simulink model "LaptopTest"  (R2015b)
settings: Solver=VariableStepAuto  StartTime=0.0  StopTime=inf  RelTol=1e-3
libraries: aerolibanimutils x1, simulink x1, dspnetwork x1
(part 1 of 4)
settings Model: Creator=Ryuu  LastModifiedBy=Ryuu

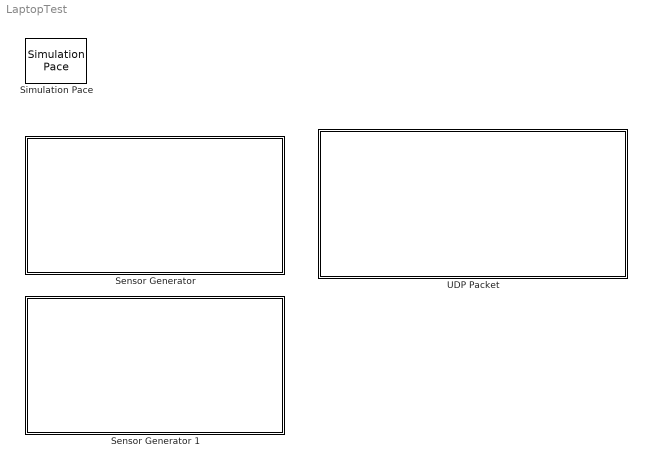
== system LaptopTest ==
  "Sensor Generator " : Subsystem
  Sensor Generator 1 : Subsystem
  Simulation Pace : aerolibanimutils/Simulation Pace  SimulationPace=1  SleepMode=MATLAB Thread  OutputPaceError=off  SampleTime=1/30
  UDP Packet : Subsystem

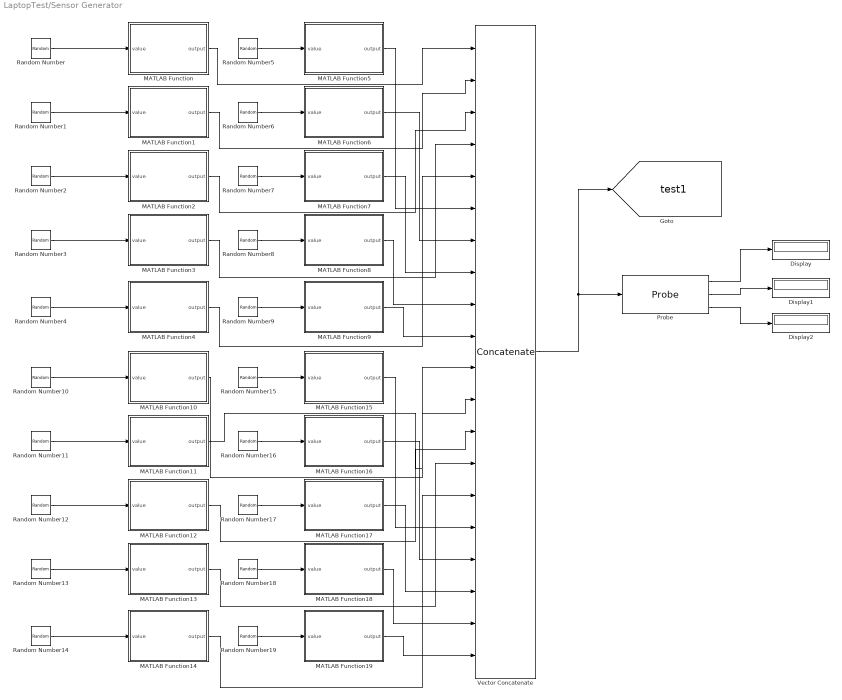
== system LaptopTest/Sensor Generator  ==
  Display : Display
  Display1 : Display
  Display2 : Display
  MATLAB Function : MATLAB Function  TreatAsAtomicUnit=on  mask(Signal Serializer){identifier=101}
      mask prompts: identifier "ID:"
      mask help:
      | Define and serialize a signal.
      |
      | The ID is the identifier of a signal.
      | - It must be unique.
      | - It must be numeric.
      | - It must match the ID defined for the signal on the GUI side.
  MATLAB Function1 : MATLAB Function  TreatAsAtomicUnit=on  mask(Signal Serializer){identifier=102}
      mask prompts: identifier "ID:"
      mask help:
      | Define and serialize a signal.
      |
      | The ID is the identifier of a signal.
      | - It must be unique.
      | - It must be numeric.
      | - It must match the ID defined for the signal on the GUI side.
  MATLAB Function10 : MATLAB Function  TreatAsAtomicUnit=on  mask(Signal Serializer){identifier=301}
      mask prompts: identifier "ID:"
      mask help:
      | Define and serialize a signal.
      |
      | The ID is the identifier of a signal.
      | - It must be unique.
      | - It must be numeric.
      | - It must match the ID defined for the signal on the GUI side.
  MATLAB Function11 : MATLAB Function  TreatAsAtomicUnit=on  mask(Signal Serializer){identifier=302}
      mask prompts: identifier "ID:"
      mask help:
      | Define and serialize a signal.
      |
      | The ID is the identifier of a signal.
      | - It must be unique.
      | - It must be numeric.
      | - It must match the ID defined for the signal on the GUI side.
  MATLAB Function12 : MATLAB Function  TreatAsAtomicUnit=on  mask(Signal Serializer){identifier=303}
      mask prompts: identifier "ID:"
      mask help:
      | Define and serialize a signal.
      |
      | The ID is the identifier of a signal.
      | - It must be unique.
      | - It must be numeric.
      | - It must match the ID defined for the signal on the GUI side.
  MATLAB Function13 : MATLAB Function  TreatAsAtomicUnit=on  mask(Signal Serializer){identifier=304}
      mask prompts: identifier "ID:"
      mask help:
      | Define and serialize a signal.
      |
      | The ID is the identifier of a signal.
      | - It must be unique.
      | - It must be numeric.
      | - It must match the ID defined for the signal on the GUI side.
  MATLAB Function14 : MATLAB Function  TreatAsAtomicUnit=on  mask(Signal Serializer){identifier=305}
      mask prompts: identifier "ID:"
      mask help:
      | Define and serialize a signal.
      |
      | The ID is the identifier of a signal.
      | - It must be unique.
      | - It must be numeric.
      | - It must match the ID defined for the signal on the GUI side.
  MATLAB Function15 : MATLAB Function  TreatAsAtomicUnit=on  mask(Signal Serializer){identifier=401}
      mask prompts: identifier "ID:"
      mask help:
      | Define and serialize a signal.
      |
      | The ID is the identifier of a signal.
      | - It must be unique.
      | - It must be numeric.
      | - It must match the ID defined for the signal on the GUI side.
  MATLAB Function16 : MATLAB Function  TreatAsAtomicUnit=on  mask(Signal Serializer){identifier=402}
      mask prompts: identifier "ID:"
      mask help:
      | Define and serialize a signal.
      |
      | The ID is the identifier of a signal.
      | - It must be unique.
      | - It must be numeric.
      | - It must match the ID defined for the signal on the GUI side.
  MATLAB Function17 : MATLAB Function  TreatAsAtomicUnit=on  mask(Signal Serializer){identifier=403}
      mask prompts: identifier "ID:"
      mask help:
      | Define and serialize a signal.
      |
      | The ID is the identifier of a signal.
      | - It must be unique.
      | - It must be numeric.
      | - It must match the ID defined for the signal on the GUI side.
  MATLAB Function18 : MATLAB Function  TreatAsAtomicUnit=on  mask(Signal Serializer){identifier=404}
      mask prompts: identifier "ID:"
      mask help:
      | Define and serialize a signal.
      |
      | The ID is the identifier of a signal.
      | - It must be unique.
      | - It must be numeric.
      | - It must match the ID defined for the signal on the GUI side.
  MATLAB Function19 : MATLAB Function  TreatAsAtomicUnit=on  mask(Signal Serializer){identifier=405}
      mask prompts: identifier "ID:"
      mask help:
      | Define and serialize a signal.
      |
      | The ID is the identifier of a signal.
      | - It must be unique.
      | - It must be numeric.
      | - It must match the ID defined for the signal on the GUI side.
  MATLAB Function2 : MATLAB Function  TreatAsAtomicUnit=on  mask(Signal Serializer){identifier=103}
      mask prompts: identifier "ID:"
      mask help:
      | Define and serialize a signal.
      |
      | The ID is the identifier of a signal.
      | - It must be unique.
      | - It must be numeric.
      | - It must match the ID defined for the signal on the GUI side.
  MATLAB Function3 : MATLAB Function  TreatAsAtomicUnit=on  mask(Signal Serializer){identifier=104}
      mask prompts: identifier "ID:"
      mask help:
      | Define and serialize a signal.
      |
      | The ID is the identifier of a signal.
      | - It must be unique.
      | - It must be numeric.
      | - It must match the ID defined for the signal on the GUI side.
  MATLAB Function4 : MATLAB Function  TreatAsAtomicUnit=on  mask(Signal Serializer){identifier=105}
      mask prompts: identifier "ID:"
      mask help:
      | Define and serialize a signal.
      |
      | The ID is the identifier of a signal.
      | - It must be unique.
      | - It must be numeric.
      | - It must match the ID defined for the signal on the GUI side.
  MATLAB Function5 : MATLAB Function  TreatAsAtomicUnit=on  mask(Signal Serializer){identifier=201}
      mask prompts: identifier "ID:"
      mask help:
      | Define and serialize a signal.
      |
      | The ID is the identifier of a signal.
      | - It must be unique.
      | - It must be numeric.
      | - It must match the ID defined for the signal on the GUI side.
  MATLAB Function6 : MATLAB Function  TreatAsAtomicUnit=on  mask(Signal Serializer){identifier=202}
      mask prompts: identifier "ID:"
      mask help:
      | Define and serialize a signal.
      |
      | The ID is the identifier of a signal.
      | - It must be unique.
      | - It must be numeric.
      | - It must match the ID defined for the signal on the GUI side.
  MATLAB Function7 : MATLAB Function  TreatAsAtomicUnit=on  mask(Signal Serializer){identifier=203}
      mask prompts: identifier "ID:"
      mask help:
      | Define and serialize a signal.
      |
      | The ID is the identifier of a signal.
      | - It must be unique.
      | - It must be numeric.
      | - It must match the ID defined for the signal on the GUI side.
  MATLAB Function8 : MATLAB Function  TreatAsAtomicUnit=on  mask(Signal Serializer){identifier=204}
      mask prompts: identifier "ID:"
      mask help:
      | Define and serialize a signal.
      |
      | The ID is the identifier of a signal.
      | - It must be unique.
      | - It must be numeric.
      | - It must match the ID defined for the signal on the GUI side.
  MATLAB Function9 : MATLAB Function  TreatAsAtomicUnit=on  mask(Signal Serializer){identifier=205}
      mask prompts: identifier "ID:"
      mask help:
      | Define and serialize a signal.
      |
      | The ID is the identifier of a signal.
      | - It must be unique.
      | - It must be numeric.
      | - It must match the ID defined for the signal on the GUI side.
  Probe : Probe  ProbeComplexSignal=off  ProbeSignalDimensions=on
  Random Number : RandomNumber  Mean=100  Variance=50  Seed=101  SampleTime=0.02
  Random Number1 : RandomNumber  Mean=100  Variance=50  Seed=102  SampleTime=0.02
  Random Number10 : RandomNumber  Mean=100  Variance=50  Seed=301  SampleTime=0.02
  Random Number11 : RandomNumber  Mean=100  Variance=50  Seed=302  SampleTime=0.02
  Random Number12 : RandomNumber  Mean=100  Variance=50  Seed=303  SampleTime=0.02
  Random Number13 : RandomNumber  Mean=100  Variance=50  Seed=304  SampleTime=0.02
  Random Number14 : RandomNumber  Mean=100  Variance=50  Seed=305  SampleTime=0.02
  Random Number15 : RandomNumber  Mean=100  Variance=50  Seed=401  SampleTime=0.02
  Random Number16 : RandomNumber  Mean=100  Variance=50  Seed=402  SampleTime=0.02
  Random Number17 : RandomNumber  Mean=100  Variance=50  Seed=403  SampleTime=0.02
  Random Number18 : RandomNumber  Mean=100  Variance=50  Seed=404  SampleTime=0.02
  Random Number19 : RandomNumber  Mean=100  Variance=50  Seed=405  SampleTime=0.02
  Random Number2 : RandomNumber  Mean=100  Variance=50  Seed=103  SampleTime=0.02
  Random Number3 : RandomNumber  Mean=100  Variance=50  Seed=104  SampleTime=0.02
  Random Number4 : RandomNumber  Mean=100  Variance=50  Seed=105  SampleTime=0.02
  Random Number5 : RandomNumber  Mean=100  Variance=50  Seed=201  SampleTime=0.02
  Random Number6 : RandomNumber  Mean=100  Variance=50  Seed=202  SampleTime=0.02
  Random Number7 : RandomNumber  Mean=100  Variance=50  Seed=203  SampleTime=0.02
  Random Number8 : RandomNumber  Mean=100  Variance=50  Seed=204  SampleTime=0.02
  Random Number9 : RandomNumber  Mean=100  Variance=50  Seed=205  SampleTime=0.02
  Vector Concatenate : Concatenate  NumInputs=20
  tag scope: test1=global
  wires:
  MATLAB Function/1(output) -> Vector Concatenate/1
  Random Number2/1 -> MATLAB Function2/1(value)
  Random Number3/1 -> MATLAB Function3/1(value)
  Random Number4/1 -> MATLAB Function4/1(value)
  Random Number5/1 -> MATLAB Function5/1(value)
  Random Number6/1 -> MATLAB Function6/1(value)
  Random Number7/1 -> MATLAB Function7/1(value)
  Random Number8/1 -> MATLAB Function8/1(value)
  Random Number9/1 -> MATLAB Function9/1(value)
  MATLAB Function1/1(output) -> Vector Concatenate/2
  MATLAB Function2/1(output) -> Vector Concatenate/3
  MATLAB Function3/1(output) -> Vector Concatenate/4
  MATLAB Function4/1(output) -> Vector Concatenate/5
  MATLAB Function5/1(output) -> Vector Concatenate/6
  MATLAB Function6/1(output) -> Vector Concatenate/7
  MATLAB Function8/1(output) -> Vector Concatenate/9
  MATLAB Function7/1(output) -> Vector Concatenate/8
  MATLAB Function9/1(output) -> Vector Concatenate/10
  Random Number/1 -> MATLAB Function/1(value)
  Random Number1/1 -> MATLAB Function1/1(value)
  Vector Concatenate/1 -> [test1], Probe/1
  Probe/1 -> Display/1
  Probe/2 -> Display1/1
  Probe/3 -> Display2/1
  MATLAB Function10/1(output) -> Vector Concatenate/11
  Random Number12/1 -> MATLAB Function12/1(value)
  Random Number13/1 -> MATLAB Function13/1(value)
  Random Number14/1 -> MATLAB Function14/1(value)
  Random Number15/1 -> MATLAB Function15/1(value)
  Random Number16/1 -> MATLAB Function16/1(value)
  Random Number17/1 -> MATLAB Function17/1(value)
  Random Number18/1 -> MATLAB Function18/1(value)
  Random Number19/1 -> MATLAB Function19/1(value)
  MATLAB Function11/1(output) -> Vector Concatenate/12
  MATLAB Function12/1(output) -> Vector Concatenate/13
  MATLAB Function13/1(output) -> Vector Concatenate/14
  MATLAB Function14/1(output) -> Vector Concatenate/15
  MATLAB Function15/1(output) -> Vector Concatenate/16
  MATLAB Function16/1(output) -> Vector Concatenate/17
  MATLAB Function18/1(output) -> Vector Concatenate/19
  MATLAB Function17/1(output) -> Vector Concatenate/18
  MATLAB Function19/1(output) -> Vector Concatenate/20
  Random Number10/1 -> MATLAB Function10/1(value)
  Random Number11/1 -> MATLAB Function11/1(value)

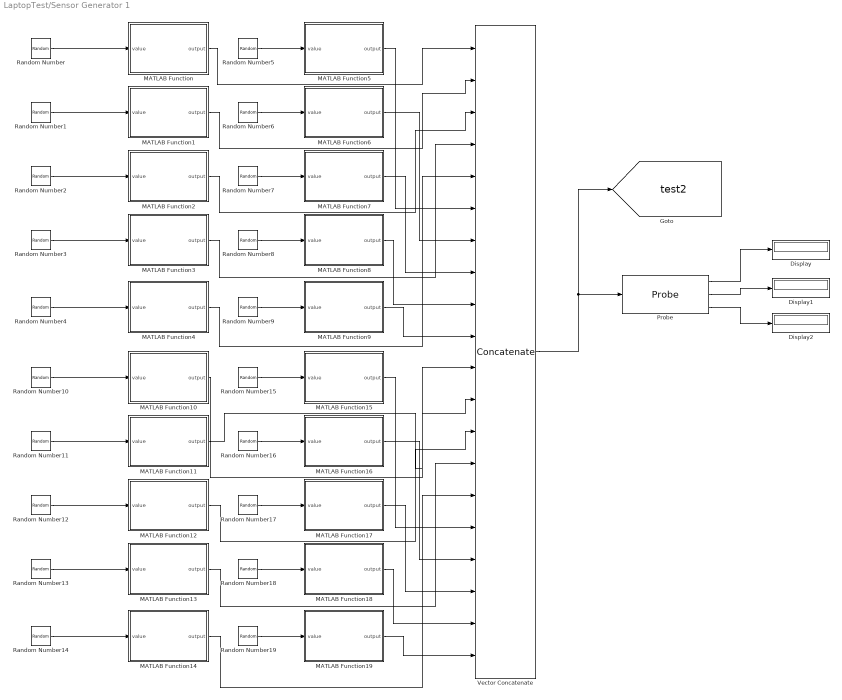
== system LaptopTest/Sensor Generator 1 ==
  Display : Display
  Display1 : Display
  Display2 : Display
  MATLAB Function : MATLAB Function  TreatAsAtomicUnit=on  mask(Signal Serializer){identifier=501}
      mask prompts: identifier "ID:"
      mask help:
      | Define and serialize a signal.
      |
      | The ID is the identifier of a signal.
      | - It must be unique.
      | - It must be numeric.
      | - It must match the ID defined for the signal on the GUI side.
  MATLAB Function1 : MATLAB Function  TreatAsAtomicUnit=on  mask(Signal Serializer){identifier=502}
      mask prompts: identifier "ID:"
      mask help:
      | Define and serialize a signal.
      |
      | The ID is the identifier of a signal.
      | - It must be unique.
      | - It must be numeric.
      | - It must match the ID defined for the signal on the GUI side.
  MATLAB Function10 : MATLAB Function  TreatAsAtomicUnit=on  mask(Signal Serializer){identifier=701}
      mask prompts: identifier "ID:"
      mask help:
      | Define and serialize a signal.
      |
      | The ID is the identifier of a signal.
      | - It must be unique.
      | - It must be numeric.
      | - It must match the ID defined for the signal on the GUI side.
  MATLAB Function11 : MATLAB Function  TreatAsAtomicUnit=on  mask(Signal Serializer){identifier=702}
      mask prompts: identifier "ID:"
      mask help:
      | Define and serialize a signal.
      |
      | The ID is the identifier of a signal.
      | - It must be unique.
      | - It must be numeric.
      | - It must match the ID defined for the signal on the GUI side.
  MATLAB Function12 : MATLAB Function  TreatAsAtomicUnit=on  mask(Signal Serializer){identifier=703}
      mask prompts: identifier "ID:"
      mask help:
      | Define and serialize a signal.
      |
      | The ID is the identifier of a signal.
      | - It must be unique.
      | - It must be numeric.
      | - It must match the ID defined for the signal on the GUI side.
  MATLAB Function13 : MATLAB Function  TreatAsAtomicUnit=on  mask(Signal Serializer){identifier=704}
      mask prompts: identifier "ID:"
      mask help:
      | Define and serialize a signal.
      |
      | The ID is the identifier of a signal.
      | - It must be unique.
      | - It must be numeric.
      | - It must match the ID defined for the signal on the GUI side.
  MATLAB Function14 : MATLAB Function  TreatAsAtomicUnit=on  mask(Signal Serializer){identifier=705}
      mask prompts: identifier "ID:"
      mask help:
      | Define and serialize a signal.
      |
      | The ID is the identifier of a signal.
      | - It must be unique.
      | - It must be numeric.
      | - It must match the ID defined for the signal on the GUI side.
  MATLAB Function15 : MATLAB Function  TreatAsAtomicUnit=on  mask(Signal Serializer){identifier=801}
      mask prompts: identifier "ID:"
      mask help:
      | Define and serialize a signal.
      |
      | The ID is the identifier of a signal.
      | - It must be unique.
      | - It must be numeric.
      | - It must match the ID defined for the signal on the GUI side.
  MATLAB Function16 : MATLAB Function  TreatAsAtomicUnit=on  mask(Signal Serializer){identifier=802}
      mask prompts: identifier "ID:"
      mask help:
      | Define and serialize a signal.
      |
      | The ID is the identifier of a signal.
      | - It must be unique.
      | - It must be numeric.
      | - It must match the ID defined for the signal on the GUI side.
  MATLAB Function17 : MATLAB Function  TreatAsAtomicUnit=on  mask(Signal Serializer){identifier=803}
      mask prompts: identifier "ID:"
      mask help:
      | Define and serialize a signal.
      |
      | The ID is the identifier of a signal.
      | - It must be unique.
      | - It must be numeric.
      | - It must match the ID defined for the signal on the GUI side.
  MATLAB Function18 : MATLAB Function  TreatAsAtomicUnit=on  mask(Signal Serializer){identifier=804}
      mask prompts: identifier "ID:"
      mask help:
      | Define and serialize a signal.
      |
      | The ID is the identifier of a signal.
      | - It must be unique.
      | - It must be numeric.
      | - It must match the ID defined for the signal on the GUI side.
  MATLAB Function19 : MATLAB Function  TreatAsAtomicUnit=on  mask(Signal Serializer){identifier=805}
      mask prompts: identifier "ID:"
      mask help:
      | Define and serialize a signal.
      |
      | The ID is the identifier of a signal.
      | - It must be unique.
      | - It must be numeric.
      | - It must match the ID defined for the signal on the GUI side.
  MATLAB Function2 : MATLAB Function  TreatAsAtomicUnit=on  mask(Signal Serializer){identifier=503}
      mask prompts: identifier "ID:"
      mask help:
      | Define and serialize a signal.
      |
      | The ID is the identifier of a signal.
      | - It must be unique.
      | - It must be numeric.
      | - It must match the ID defined for the signal on the GUI side.
  MATLAB Function3 : MATLAB Function  TreatAsAtomicUnit=on  mask(Signal Serializer){identifier=504}
      mask prompts: identifier "ID:"
      mask help:
      | Define and serialize a signal.
      |
      | The ID is the identifier of a signal.
      | - It must be unique.
      | - It must be numeric.
      | - It must match the ID defined for the signal on the GUI side.
  MATLAB Function4 : MATLAB Function  TreatAsAtomicUnit=on  mask(Signal Serializer){identifier=505}
      mask prompts: identifier "ID:"
      mask help:
      | Define and serialize a signal.
      |
      | The ID is the identifier of a signal.
      | - It must be unique.
      | - It must be numeric.
      | - It must match the ID defined for the signal on the GUI side.
  MATLAB Function5 : MATLAB Function  TreatAsAtomicUnit=on  mask(Signal Serializer){identifier=601}
      mask prompts: identifier "ID:"
      mask help:
      | Define and serialize a signal.
      |
      | The ID is the identifier of a signal.
      | - It must be unique.
      | - It must be numeric.
      | - It must match the ID defined for the signal on the GUI side.
  MATLAB Function6 : MATLAB Function  TreatAsAtomicUnit=on  mask(Signal Serializer){identifier=602}
      mask prompts: identifier "ID:"
      mask help:
      | Define and serialize a signal.
      |
      | The ID is the identifier of a signal.
      | - It must be unique.
      | - It must be numeric.
      | - It must match the ID defined for the signal on the GUI side.
  MATLAB Function7 : MATLAB Function  TreatAsAtomicUnit=on  mask(Signal Serializer){identifier=603}
      mask prompts: identifier "ID:"
      mask help:
      | Define and serialize a signal.
      |
      | The ID is the identifier of a signal.
      | - It must be unique.
      | - It must be numeric.
      | - It must match the ID defined for the signal on the GUI side.
  MATLAB Function8 : MATLAB Function  TreatAsAtomicUnit=on  mask(Signal Serializer){identifier=604}
      mask prompts: identifier "ID:"
      mask help:
      | Define and serialize a signal.
      |
      | The ID is the identifier of a signal.
      | - It must be unique.
      | - It must be numeric.
      | - It must match the ID defined for the signal on the GUI side.
  MATLAB Function9 : MATLAB Function  TreatAsAtomicUnit=on  mask(Signal Serializer){identifier=605}
      mask prompts: identifier "ID:"
      mask help:
      | Define and serialize a signal.
      |
      | The ID is the identifier of a signal.
      | - It must be unique.
      | - It must be numeric.
      | - It must match the ID defined for the signal on the GUI side.
  Probe : Probe  ProbeComplexSignal=off  ProbeSignalDimensions=on
  Random Number : RandomNumber  Mean=100  Variance=50  Seed=501  SampleTime=0.02
  Random Number1 : RandomNumber  Mean=100  Variance=50  Seed=502  SampleTime=0.02
  Random Number10 : RandomNumber  Mean=100  Variance=50  Seed=701  SampleTime=0.02
  Random Number11 : RandomNumber  Mean=100  Variance=50  Seed=702  SampleTime=0.02
  Random Number12 : RandomNumber  Mean=100  Variance=50  Seed=703  SampleTime=0.02
  Random Number13 : RandomNumber  Mean=100  Variance=50  Seed=704  SampleTime=0.02
  Random Number14 : RandomNumber  Mean=100  Variance=50  Seed=705  SampleTime=0.02
  Random Number15 : RandomNumber  Mean=100  Variance=50  Seed=801  SampleTime=0.02
  Random Number16 : RandomNumber  Mean=100  Variance=50  Seed=802  SampleTime=0.02
  Random Number17 : RandomNumber  Mean=100  Variance=50  Seed=803  SampleTime=0.02
  Random Number18 : RandomNumber  Mean=100  Variance=50  Seed=804  SampleTime=0.02
  Random Number19 : RandomNumber  Mean=100  Variance=50  Seed=805  SampleTime=0.02
  Random Number2 : RandomNumber  Mean=100  Variance=50  Seed=503  SampleTime=0.02
  Random Number3 : RandomNumber  Mean=100  Variance=50  Seed=504  SampleTime=0.02
  Random Number4 : RandomNumber  Mean=100  Variance=50  Seed=505  SampleTime=0.02
  Random Number5 : RandomNumber  Mean=100  Variance=50  Seed=601  SampleTime=0.02
  Random Number6 : RandomNumber  Mean=100  Variance=50  Seed=602  SampleTime=0.02
  Random Number7 : RandomNumber  Mean=100  Variance=50  Seed=603  SampleTime=0.02
  Random Number8 : RandomNumber  Mean=100  Variance=50  Seed=604  SampleTime=0.02
  Random Number9 : RandomNumber  Mean=100  Variance=50  Seed=605  SampleTime=0.02
  Vector Concatenate : Concatenate  NumInputs=20
  tag scope: test2=global
  wires:
  MATLAB Function/1(output) -> Vector Concatenate/1
  Random Number2/1 -> MATLAB Function2/1(value)
  Random Number3/1 -> MATLAB Function3/1(value)
  Random Number4/1 -> MATLAB Function4/1(value)
  Random Number5/1 -> MATLAB Function5/1(value)
  Random Number6/1 -> MATLAB Function6/1(value)
  Random Number7/1 -> MATLAB Function7/1(value)
  Random Number8/1 -> MATLAB Function8/1(value)
  Random Number9/1 -> MATLAB Function9/1(value)
  MATLAB Function1/1(output) -> Vector Concatenate/2
  MATLAB Function2/1(output) -> Vector Concatenate/3
  MATLAB Function3/1(output) -> Vector Concatenate/4
  MATLAB Function4/1(output) -> Vector Concatenate/5
  MATLAB Function5/1(output) -> Vector Concatenate/6
  MATLAB Function6/1(output) -> Vector Concatenate/7
  MATLAB Function8/1(output) -> Vector Concatenate/9
  MATLAB Function7/1(output) -> Vector Concatenate/8
  MATLAB Function9/1(output) -> Vector Concatenate/10
  Random Number/1 -> MATLAB Function/1(value)
  Random Number1/1 -> MATLAB Function1/1(value)
  Vector Concatenate/1 -> [test2], Probe/1
  Probe/1 -> Display/1
  Probe/2 -> Display1/1
  Probe/3 -> Display2/1
  MATLAB Function10/1(output) -> Vector Concatenate/11
  Random Number12/1 -> MATLAB Function12/1(value)
  Random Number13/1 -> MATLAB Function13/1(value)
  Random Number14/1 -> MATLAB Function14/1(value)
  Random Number15/1 -> MATLAB Function15/1(value)
  Random Number16/1 -> MATLAB Function16/1(value)
  Random Number17/1 -> MATLAB Function17/1(value)
  Random Number18/1 -> MATLAB Function18/1(value)
  Random Number19/1 -> MATLAB Function19/1(value)
  MATLAB Function11/1(output) -> Vector Concatenate/12
  MATLAB Function12/1(output) -> Vector Concatenate/13
  MATLAB Function13/1(output) -> Vector Concatenate/14
  MATLAB Function14/1(output) -> Vector Concatenate/15
  MATLAB Function15/1(output) -> Vector Concatenate/16
  MATLAB Function16/1(output) -> Vector Concatenate/17
  MATLAB Function18/1(output) -> Vector Concatenate/19
  MATLAB Function17/1(output) -> Vector Concatenate/18
  MATLAB Function19/1(output) -> Vector Concatenate/20
  Random Number10/1 -> MATLAB Function10/1(value)
  Random Number11/1 -> MATLAB Function11/1(value)

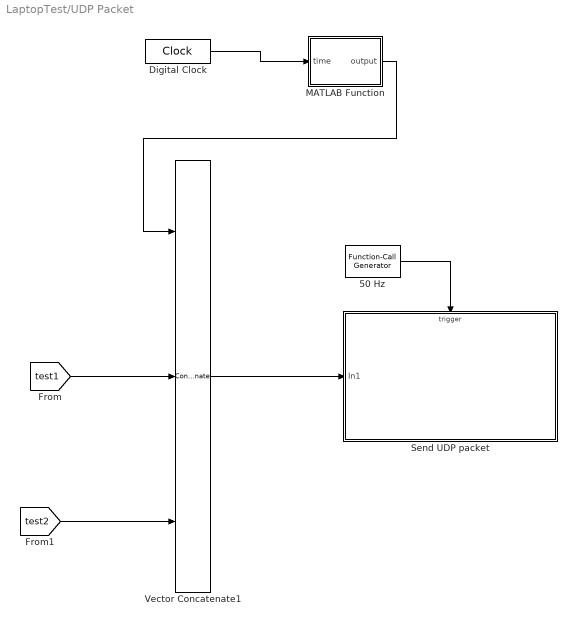
== system LaptopTest/UDP Packet ==
  50 Hz : simulink/Ports & Subsystems/Function-Call Generator  sample_time=0.02  numberOfIterations=1
  Digital Clock : DigitalClock  SampleTime=0.001
  MATLAB Function : MATLAB Function  TreatAsAtomicUnit=on
  Send UDP packet : Subsystem
  Vector Concatenate1 : Concatenate  NumInputs=3
  wires:
  [test1] -> Vector Concatenate1/2
  50 Hz/1 -> Send UDP packet/Trigger
  Vector Concatenate1/1 -> Send UDP packet/1(In1)
  Digital Clock/1 -> MATLAB Function/1(time)
  MATLAB Function/1(output) -> Vector Concatenate1/1
  [test2] -> Vector Concatenate1/3

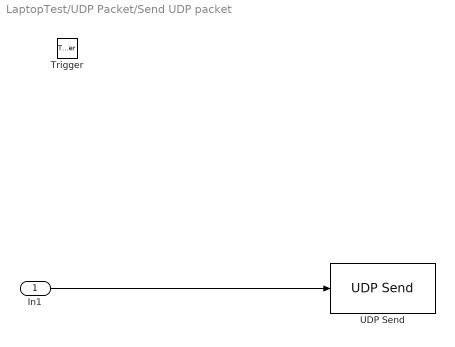
== system LaptopTest/UDP Packet/Send UDP packet ==
  In1 : Inport
  Trigger : TriggerPort  TriggerType=function-call  PortDimensions=1
  UDP Send : dspnetwork/UDP Send  remoteURL='192.168.21.1'  remotePort=25000  localURL='0.0.0.0'  localPortSource=Automatically determine  localPort=-1  sampletime=-1  separateLengthPort=0
  wires:
  In1/1 -> UDP Send/1

== matlab function LaptopTest/Sensor Generator /MATLAB Function1 ==
  data: value input; output output uint8 size=18; identifier parameter double
function output = data_serialize(value, identifier)

id_ser = sensor_serialize(identifier);
value_ser = sensor_serialize(value);

output = [
    id_ser;
    value_ser;
    ];
end


function m = sensor_serialize(v)
    % dispatch according to type
    if isnumeric(v) 
        m = serialize_numeric(v);
    elseif ischar(v)
        m = serialize_string(v);
    elseif islogical(v)
        m = serialize_logical(v);
	else
		error('Unsupported data type');
    end
end

% single scalar
function m = serialize_scalar(v)
    % Data type & data
    m = [class2tag(class(v)); typecast(v,'uint8').'];
end

% char arrays
function m = serialize_string(v)
    if size(v,1) == 1
        % horizontal string: Type, Length, and Data
        m = [uint8(0); typecast(uint32(length(v)),'uint8').'; uint8(v(:))];
    elseif sum(size(v)) == 0
        % '': special encoding
        m = uint8(200);
    else
        % general char array: Tag & Number of dimensions, Dimensions, Data
        m = [uint8(132); ndims(v); typecast(uint32(size(v)),'uint8').'; uint8(v(:))];
    end
end

% logical arrays
function m = serialize_logical(v)
    % Tag & Number of dimensions, Dimensions, Data
    m = [uint8(133); ndims(v); typecast(uint32(size(v)),'uint8').'; uint8(v(:))];
end

% non-complex and non-sparse numerical matrix
function m = serialize_numeric_simple(v)
    % Tag & Number of dimensions, Dimensions, Data
    m = [16+class2tag(class(v)); ndims(v); typecast(uint32(size(v)),'uint8').'; typecast(v(:).','uint8').'];
end

% Numeric Matrix: can be real/complex, sparse/full, scalar
function m = serialize_numeric(v)
    if issparse(v)
        % Data Type & Dimensions
        m = [uint8(130); typecast(uint64(size(v,1)), 'uint8').'; typecast(uint64(size(v,2)), 'uint8').']; % vectorize
        % Index vectors
        [i,j,s] = find(v);        
        % Real/Complex
        if isreal(v)
            m = [m; serialize_numeric_simple(i); serialize_numeric_simple(j); 1; serialize_numeric_simple(s)];
        else
            m = [m; serialize_numeric_simple(i); serialize_numeric_simple(j); 0; serialize_numeric_simple(real(s)); serialize_numeric_simple(imag(s))];
        end
    elseif ~isreal(v)
        % Data type & contents
        m = [uint8(131); serialize_numeric_simple(real(v)); serialize_numeric_simple(imag(v))];
    elseif isscalar(v)
        % Scalar
        m = serialize_scalar(v);
    else
        % Simple matrix
        m = serialize_numeric_simple(v);
    end
end

% *container* class to byte
function b = class2tag(cls)
	switch cls
		case 'string'
            b = uint8(0);
		case 'double'
			b = uint8(1);
		case 'single'
			b = uint8(2);
		case 'int8'
			b = uint8(3);
		case 'uint8'
			b = uint8(4);
		case 'int16'
			b = uint8(5);
		case 'uint16'
			b = uint8(6);
		case 'int32'
			b = uint8(7);
		case 'uint32'
			b = uint8(8);
		case 'int64'
			b = uint8(9);
		case 'uint64'
			b = uint8(10);
		otherwise
			error('Unknown class');
    end
end

== matlab function LaptopTest/Sensor Generator /MATLAB Function ==
  data: value input; output output uint8 size=18; identifier parameter double
function output = data_serialize(value, identifier)

id_ser = sensor_serialize(identifier);
value_ser = sensor_serialize(value);

output = [
    id_ser;
    value_ser;
    ];
end


function m = sensor_serialize(v)
    % dispatch according to type
    if isnumeric(v) 
        m = serialize_numeric(v);
    elseif ischar(v)
        m = serialize_string(v);
    elseif islogical(v)
        m = serialize_logical(v);
	else
		error('Unsupported data type');
    end
end

% single scalar
function m = serialize_scalar(v)
    % Data type & data
    m = [class2tag(class(v)); typecast(v,'uint8').'];
end

% char arrays
function m = serialize_string(v)
    if size(v,1) == 1
        % horizontal string: Type, Length, and Data
        m = [uint8(0); typecast(uint32(length(v)),'uint8').'; uint8(v(:))];
    elseif sum(size(v)) == 0
        % '': special encoding
        m = uint8(200);
    else
        % general char array: Tag & Number of dimensions, Dimensions, Data
        m = [uint8(132); ndims(v); typecast(uint32(size(v)),'uint8').'; uint8(v(:))];
    end
end

% logical arrays
function m = serialize_logical(v)
    % Tag & Number of dimensions, Dimensions, Data
    m = [uint8(133); ndims(v); typecast(uint32(size(v)),'uint8').'; uint8(v(:))];
end

% non-complex and non-sparse numerical matrix
function m = serialize_numeric_simple(v)
    % Tag & Number of dimensions, Dimensions, Data
    m = [16+class2tag(class(v)); ndims(v); typecast(uint32(size(v)),'uint8').'; typecast(v(:).','uint8').'];
end

% Numeric Matrix: can be real/complex, sparse/full, scalar
function m = serialize_numeric(v)
    if issparse(v)
        % Data Type & Dimensions
        m = [uint8(130); typecast(uint64(size(v,1)), 'uint8').'; typecast(uint64(size(v,2)), 'uint8').']; % vectorize
        % Index vectors
        [i,j,s] = find(v);        
        % Real/Complex
        if isreal(v)
            m = [m; serialize_numeric_simple(i); serialize_numeric_simple(j); 1; serialize_numeric_simple(s)];
        else
            m = [m; serialize_numeric_simple(i); serialize_numeric_simple(j); 0; serialize_numeric_simple(real(s)); serialize_numeric_simple(imag(s))];
        end
    elseif ~isreal(v)
        % Data type & contents
        m = [uint8(131); serialize_numeric_simple(real(v)); serialize_numeric_simple(imag(v))];
    elseif isscalar(v)
        % Scalar
        m = serialize_scalar(v);
    else
        % Simple matrix
        m = serialize_numeric_simple(v);
    end
end

% *container* class to byte
function b = class2tag(cls)
	switch cls
		case 'string'
            b = uint8(0);
		case 'double'
			b = uint8(1);
		case 'single'
			b = uint8(2);
		case 'int8'
			b = uint8(3);
		case 'uint8'
			b = uint8(4);
		case 'int16'
			b = uint8(5);
		case 'uint16'
			b = uint8(6);
		case 'int32'
			b = uint8(7);
		case 'uint32'
			b = uint8(8);
		case 'int64'
			b = uint8(9);
		case 'uint64'
			b = uint8(10);
		otherwise
			error('Unknown class');
    end
end

== matlab function LaptopTest/Sensor Generator /MATLAB Function2 ==
  data: value input; output output uint8 size=18; identifier parameter double
function output = data_serialize(value, identifier)

id_ser = sensor_serialize(identifier);
value_ser = sensor_serialize(value);

output = [
    id_ser;
    value_ser;
    ];
end


function m = sensor_serialize(v)
    % dispatch according to type
    if isnumeric(v) 
        m = serialize_numeric(v);
    elseif ischar(v)
        m = serialize_string(v);
    elseif islogical(v)
        m = serialize_logical(v);
	else
		error('Unsupported data type');
    end
end

% single scalar
function m = serialize_scalar(v)
    % Data type & data
    m = [class2tag(class(v)); typecast(v,'uint8').'];
end

% char arrays
function m = serialize_string(v)
    if size(v,1) == 1
        % horizontal string: Type, Length, and Data
        m = [uint8(0); typecast(uint32(length(v)),'uint8').'; uint8(v(:))];
    elseif sum(size(v)) == 0
        % '': special encoding
        m = uint8(200);
    else
        % general char array: Tag & Number of dimensions, Dimensions, Data
        m = [uint8(132); ndims(v); typecast(uint32(size(v)),'uint8').'; uint8(v(:))];
    end
end

% logical arrays
function m = serialize_logical(v)
    % Tag & Number of dimensions, Dimensions, Data
    m = [uint8(133); ndims(v); typecast(uint32(size(v)),'uint8').'; uint8(v(:))];
end

% non-complex and non-sparse numerical matrix
function m = serialize_numeric_simple(v)
    % Tag & Number of dimensions, Dimensions, Data
    m = [16+class2tag(class(v)); ndims(v); typecast(uint32(size(v)),'uint8').'; typecast(v(:).','uint8').'];
end

% Numeric Matrix: can be real/complex, sparse/full, scalar
function m = serialize_numeric(v)
    if issparse(v)
        % Data Type & Dimensions
        m = [uint8(130); typecast(uint64(size(v,1)), 'uint8').'; typecast(uint64(size(v,2)), 'uint8').']; % vectorize
        % Index vectors
        [i,j,s] = find(v);        
        % Real/Complex
        if isreal(v)
            m = [m; serialize_numeric_simple(i); serialize_numeric_simple(j); 1; serialize_numeric_simple(s)];
        else
            m = [m; serialize_numeric_simple(i); serialize_numeric_simple(j); 0; serialize_numeric_simple(real(s)); serialize_numeric_simple(imag(s))];
        end
    elseif ~isreal(v)
        % Data type & contents
        m = [uint8(131); serialize_numeric_simple(real(v)); serialize_numeric_simple(imag(v))];
    elseif isscalar(v)
        % Scalar
        m = serialize_scalar(v);
    else
        % Simple matrix
        m = serialize_numeric_simple(v);
    end
end

% *container* class to byte
function b = class2tag(cls)
	switch cls
		case 'string'
            b = uint8(0);
		case 'double'
			b = uint8(1);
		case 'single'
			b = uint8(2);
		case 'int8'
			b = uint8(3);
		case 'uint8'
			b = uint8(4);
		case 'int16'
			b = uint8(5);
		case 'uint16'
			b = uint8(6);
		case 'int32'
			b = uint8(7);
		case 'uint32'
			b = uint8(8);
		case 'int64'
			b = uint8(9);
		case 'uint64'
			b = uint8(10);
		otherwise
			error('Unknown class');
    end
end

== matlab function LaptopTest/Sensor Generator /MATLAB Function3 ==
  data: value input; output output uint8 size=18; identifier parameter double
function output = data_serialize(value, identifier)

id_ser = sensor_serialize(identifier);
value_ser = sensor_serialize(value);

output = [
    id_ser;
    value_ser;
    ];
end


function m = sensor_serialize(v)
    % dispatch according to type
    if isnumeric(v) 
        m = serialize_numeric(v);
    elseif ischar(v)
        m = serialize_string(v);
    elseif islogical(v)
        m = serialize_logical(v);
	else
		error('Unsupported data type');
    end
end

% single scalar
function m = serialize_scalar(v)
    % Data type & data
    m = [class2tag(class(v)); typecast(v,'uint8').'];
end

% char arrays
function m = serialize_string(v)
    if size(v,1) == 1
        % horizontal string: Type, Length, and Data
        m = [uint8(0); typecast(uint32(length(v)),'uint8').'; uint8(v(:))];
    elseif sum(size(v)) == 0
        % '': special encoding
        m = uint8(200);
    else
        % general char array: Tag & Number of dimensions, Dimensions, Data
        m = [uint8(132); ndims(v); typecast(uint32(size(v)),'uint8').'; uint8(v(:))];
    end
end

% logical arrays
function m = serialize_logical(v)
    % Tag & Number of dimensions, Dimensions, Data
    m = [uint8(133); ndims(v); typecast(uint32(size(v)),'uint8').'; uint8(v(:))];
end

% non-complex and non-sparse numerical matrix
function m = serialize_numeric_simple(v)
    % Tag & Number of dimensions, Dimensions, Data
    m = [16+class2tag(class(v)); ndims(v); typecast(uint32(size(v)),'uint8').'; typecast(v(:).','uint8').'];
end

% Numeric Matrix: can be real/complex, sparse/full, scalar
function m = serialize_numeric(v)
    if issparse(v)
        % Data Type & Dimensions
        m = [uint8(130); typecast(uint64(size(v,1)), 'uint8').'; typecast(uint64(size(v,2)), 'uint8').']; % vectorize
        % Index vectors
        [i,j,s] = find(v);        
        % Real/Complex
        if isreal(v)
            m = [m; serialize_numeric_simple(i); serialize_numeric_simple(j); 1; serialize_numeric_simple(s)];
        else
            m = [m; serialize_numeric_simple(i); serialize_numeric_simple(j); 0; serialize_numeric_simple(real(s)); serialize_numeric_simple(imag(s))];
        end
    elseif ~isreal(v)
        % Data type & contents
        m = [uint8(131); serialize_numeric_simple(real(v)); serialize_numeric_simple(imag(v))];
    elseif isscalar(v)
        % Scalar
        m = serialize_scalar(v);
    else
        % Simple matrix
        m = serialize_numeric_simple(v);
    end
end

% *container* class to byte
function b = class2tag(cls)
	switch cls
		case 'string'
            b = uint8(0);
		case 'double'
			b = uint8(1);
		case 'single'
			b = uint8(2);
		case 'int8'
			b = uint8(3);
		case 'uint8'
			b = uint8(4);
		case 'int16'
			b = uint8(5);
		case 'uint16'
			b = uint8(6);
		case 'int32'
			b = uint8(7);
		case 'uint32'
			b = uint8(8);
		case 'int64'
			b = uint8(9);
		case 'uint64'
			b = uint8(10);
		otherwise
			error('Unknown class');
    end
end

== matlab function LaptopTest/Sensor Generator /MATLAB Function4 ==
  data: value input; output output uint8 size=18; identifier parameter double
function output = data_serialize(value, identifier)

id_ser = sensor_serialize(identifier);
value_ser = sensor_serialize(value);

output = [
    id_ser;
    value_ser;
    ];
end


function m = sensor_serialize(v)
    % dispatch according to type
    if isnumeric(v) 
        m = serialize_numeric(v);
    elseif ischar(v)
        m = serialize_string(v);
    elseif islogical(v)
        m = serialize_logical(v);
	else
		error('Unsupported data type');
    end
end

% single scalar
function m = serialize_scalar(v)
    % Data type & data
    m = [class2tag(class(v)); typecast(v,'uint8').'];
end

% char arrays
function m = serialize_string(v)
    if size(v,1) == 1
        % horizontal string: Type, Length, and Data
        m = [uint8(0); typecast(uint32(length(v)),'uint8').'; uint8(v(:))];
    elseif sum(size(v)) == 0
        % '': special encoding
        m = uint8(200);
    else
        % general char array: Tag & Number of dimensions, Dimensions, Data
        m = [uint8(132); ndims(v); typecast(uint32(size(v)),'uint8').'; uint8(v(:))];
    end
end

% logical arrays
function m = serialize_logical(v)
    % Tag & Number of dimensions, Dimensions, Data
    m = [uint8(133); ndims(v); typecast(uint32(size(v)),'uint8').'; uint8(v(:))];
end

% non-complex and non-sparse numerical matrix
function m = serialize_numeric_simple(v)
    % Tag & Number of dimensions, Dimensions, Data
    m = [16+class2tag(class(v)); ndims(v); typecast(uint32(size(v)),'uint8').'; typecast(v(:).','uint8').'];
end

% Numeric Matrix: can be real/complex, sparse/full, scalar
function m = serialize_numeric(v)
    if issparse(v)
        % Data Type & Dimensions
        m = [uint8(130); typecast(uint64(size(v,1)), 'uint8').'; typecast(uint64(size(v,2)), 'uint8').']; % vectorize
        % Index vectors
        [i,j,s] = find(v);        
        % Real/Complex
        if isreal(v)
            m = [m; serialize_numeric_simple(i); serialize_numeric_simple(j); 1; serialize_numeric_simple(s)];
        else
            m = [m; serialize_numeric_simple(i); serialize_numeric_simple(j); 0; serialize_numeric_simple(real(s)); serialize_numeric_simple(imag(s))];
        end
    elseif ~isreal(v)
        % Data type & contents
        m = [uint8(131); serialize_numeric_simple(real(v)); serialize_numeric_simple(imag(v))];
    elseif isscalar(v)
        % Scalar
        m = serialize_scalar(v);
    else
        % Simple matrix
        m = serialize_numeric_simple(v);
    end
end

% *container* class to byte
function b = class2tag(cls)
	switch cls
		case 'string'
            b = uint8(0);
		case 'double'
			b = uint8(1);
		case 'single'
			b = uint8(2);
		case 'int8'
			b = uint8(3);
		case 'uint8'
			b = uint8(4);
		case 'int16'
			b = uint8(5);
		case 'uint16'
			b = uint8(6);
		case 'int32'
			b = uint8(7);
		case 'uint32'
			b = uint8(8);
		case 'int64'
			b = uint8(9);
		case 'uint64'
			b = uint8(10);
		otherwise
			error('Unknown class');
    end
end

== matlab function LaptopTest/Sensor Generator /MATLAB Function5 ==
  data: value input; output output uint8 size=18; identifier parameter double
function output = data_serialize(value, identifier)

id_ser = sensor_serialize(identifier);
value_ser = sensor_serialize(value);

output = [
    id_ser;
    value_ser;
    ];
end


function m = sensor_serialize(v)
    % dispatch according to type
    if isnumeric(v) 
        m = serialize_numeric(v);
    elseif ischar(v)
        m = serialize_string(v);
    elseif islogical(v)
        m = serialize_logical(v);
	else
		error('Unsupported data type');
    end
end

% single scalar
function m = serialize_scalar(v)
    % Data type & data
    m = [class2tag(class(v)); typecast(v,'uint8').'];
end

% char arrays
function m = serialize_string(v)
    if size(v,1) == 1
        % horizontal string: Type, Length, and Data
        m = [uint8(0); typecast(uint32(length(v)),'uint8').'; uint8(v(:))];
    elseif sum(size(v)) == 0
        % '': special encoding
        m = uint8(200);
    else
        % general char array: Tag & Number of dimensions, Dimensions, Data
        m = [uint8(132); ndims(v); typecast(uint32(size(v)),'uint8').'; uint8(v(:))];
    end
end

% logical arrays
function m = serialize_logical(v)
    % Tag & Number of dimensions, Dimensions, Data
    m = [uint8(133); ndims(v); typecast(uint32(size(v)),'uint8').'; uint8(v(:))];
end

% non-complex and non-sparse numerical matrix
function m = serialize_numeric_simple(v)
    % Tag & Number of dimensions, Dimensions, Data
    m = [16+class2tag(class(v)); ndims(v); typecast(uint32(size(v)),'uint8').'; typecast(v(:).','uint8').'];
end

% Numeric Matrix: can be real/complex, sparse/full, scalar
function m = serialize_numeric(v)
    if issparse(v)
        % Data Type & Dimensions
        m = [uint8(130); typecast(uint64(size(v,1)), 'uint8').'; typecast(uint64(size(v,2)), 'uint8').']; % vectorize
        % Index vectors
        [i,j,s] = find(v);        
        % Real/Complex
        if isreal(v)
            m = [m; serialize_numeric_simple(i); serialize_numeric_simple(j); 1; serialize_numeric_simple(s)];
        else
            m = [m; serialize_numeric_simple(i); serialize_numeric_simple(j); 0; serialize_numeric_simple(real(s)); serialize_numeric_simple(imag(s))];
        end
    elseif ~isreal(v)
        % Data type & contents
        m = [uint8(131); serialize_numeric_simple(real(v)); serialize_numeric_simple(imag(v))];
    elseif isscalar(v)
        % Scalar
        m = serialize_scalar(v);
    else
        % Simple matrix
        m = serialize_numeric_simple(v);
    end
end

% *container* class to byte
function b = class2tag(cls)
	switch cls
		case 'string'
            b = uint8(0);
		case 'double'
			b = uint8(1);
		case 'single'
			b = uint8(2);
		case 'int8'
			b = uint8(3);
		case 'uint8'
			b = uint8(4);
		case 'int16'
			b = uint8(5);
		case 'uint16'
			b = uint8(6);
		case 'int32'
			b = uint8(7);
		case 'uint32'
			b = uint8(8);
		case 'int64'
			b = uint8(9);
		case 'uint64'
			b = uint8(10);
		otherwise
			error('Unknown class');
    end
end

== matlab function LaptopTest/Sensor Generator /MATLAB Function6 ==
  data: value input; output output uint8 size=18; identifier parameter double
function output = data_serialize(value, identifier)

id_ser = sensor_serialize(identifier);
value_ser = sensor_serialize(value);

output = [
    id_ser;
    value_ser;
    ];
end


function m = sensor_serialize(v)
    % dispatch according to type
    if isnumeric(v) 
        m = serialize_numeric(v);
    elseif ischar(v)
        m = serialize_string(v);
    elseif islogical(v)
        m = serialize_logical(v);
	else
		error('Unsupported data type');
    end
end

% single scalar
function m = serialize_scalar(v)
    % Data type & data
    m = [class2tag(class(v)); typecast(v,'uint8').'];
end

% char arrays
function m = serialize_string(v)
    if size(v,1) == 1
        % horizontal string: Type, Length, and Data
        m = [uint8(0); typecast(uint32(length(v)),'uint8').'; uint8(v(:))];
    elseif sum(size(v)) == 0
        % '': special encoding
        m = uint8(200);
    else
        % general char array: Tag & Number of dimensions, Dimensions, Data
        m = [uint8(132); ndims(v); typecast(uint32(size(v)),'uint8').'; uint8(v(:))];
    end
end

% logical arrays
function m = serialize_logical(v)
    % Tag & Number of dimensions, Dimensions, Data
    m = [uint8(133); ndims(v); typecast(uint32(size(v)),'uint8').'; uint8(v(:))];
end

% non-complex and non-sparse numerical matrix
function m = serialize_numeric_simple(v)
    % Tag & Number of dimensions, Dimensions, Data
    m = [16+class2tag(class(v)); ndims(v); typecast(uint32(size(v)),'uint8').'; typecast(v(:).','uint8').'];
end

% Numeric Matrix: can be real/complex, sparse/full, scalar
function m = serialize_numeric(v)
    if issparse(v)
        % Data Type & Dimensions
        m = [uint8(130); typecast(uint64(size(v,1)), 'uint8').'; typecast(uint64(size(v,2)), 'uint8').']; % vectorize
        % Index vectors
        [i,j,s] = find(v);        
        % Real/Complex
        if isreal(v)
            m = [m; serialize_numeric_simple(i); serialize_numeric_simple(j); 1; serialize_numeric_simple(s)];
        else
            m = [m; serialize_numeric_simple(i); serialize_numeric_simple(j); 0; serialize_numeric_simple(real(s)); serialize_numeric_simple(imag(s))];
        end
    elseif ~isreal(v)
        % Data type & contents
        m = [uint8(131); serialize_numeric_simple(real(v)); serialize_numeric_simple(imag(v))];
    elseif isscalar(v)
        % Scalar
        m = serialize_scalar(v);
    else
        % Simple matrix
        m = serialize_numeric_simple(v);
    end
end

% *container* class to byte
function b = class2tag(cls)
	switch cls
		case 'string'
            b = uint8(0);
		case 'double'
			b = uint8(1);
		case 'single'
			b = uint8(2);
		case 'int8'
			b = uint8(3);
		case 'uint8'
			b = uint8(4);
		case 'int16'
			b = uint8(5);
		case 'uint16'
			b = uint8(6);
		case 'int32'
			b = uint8(7);
		case 'uint32'
			b = uint8(8);
		case 'int64'
			b = uint8(9);
		case 'uint64'
			b = uint8(10);
		otherwise
			error('Unknown class');
    end
end

== matlab function LaptopTest/Sensor Generator /MATLAB Function7 ==
  data: value input; output output uint8 size=18; identifier parameter double
function output = data_serialize(value, identifier)

id_ser = sensor_serialize(identifier);
value_ser = sensor_serialize(value);

output = [
    id_ser;
    value_ser;
    ];
end


function m = sensor_serialize(v)
    % dispatch according to type
    if isnumeric(v) 
        m = serialize_numeric(v);
    elseif ischar(v)
        m = serialize_string(v);
    elseif islogical(v)
        m = serialize_logical(v);
	else
		error('Unsupported data type');
    end
end

% single scalar
function m = serialize_scalar(v)
    % Data type & data
    m = [class2tag(class(v)); typecast(v,'uint8').'];
end

% char arrays
function m = serialize_string(v)
    if size(v,1) == 1
        % horizontal string: Type, Length, and Data
        m = [uint8(0); typecast(uint32(length(v)),'uint8').'; uint8(v(:))];
    elseif sum(size(v)) == 0
        % '': special encoding
        m = uint8(200);
    else
        % general char array: Tag & Number of dimensions, Dimensions, Data
        m = [uint8(132); ndims(v); typecast(uint32(size(v)),'uint8').'; uint8(v(:))];
    end
end

% logical arrays
function m = serialize_logical(v)
    % Tag & Number of dimensions, Dimensions, Data
    m = [uint8(133); ndims(v); typecast(uint32(size(v)),'uint8').'; uint8(v(:))];
end

% non-complex and non-sparse numerical matrix
function m = serialize_numeric_simple(v)
    % Tag & Number of dimensions, Dimensions, Data
    m = [16+class2tag(class(v)); ndims(v); typecast(uint32(size(v)),'uint8').'; typecast(v(:).','uint8').'];
end

% Numeric Matrix: can be real/complex, sparse/full, scalar
function m = serialize_numeric(v)
    if issparse(v)
        % Data Type & Dimensions
        m = [uint8(130); typecast(uint64(size(v,1)), 'uint8').'; typecast(uint64(size(v,2)), 'uint8').']; % vectorize
        % Index vectors
        [i,j,s] = find(v);        
        % Real/Complex
        if isreal(v)
            m = [m; serialize_numeric_simple(i); serialize_numeric_simple(j); 1; serialize_numeric_simple(s)];
        else
            m = [m; serialize_numeric_simple(i); serialize_numeric_simple(j); 0; serialize_numeric_simple(real(s)); serialize_numeric_simple(imag(s))];
        end
    elseif ~isreal(v)
        % Data type & contents
        m = [uint8(131); serialize_numeric_simple(real(v)); serialize_numeric_simple(imag(v))];
    elseif isscalar(v)
        % Scalar
        m = serialize_scalar(v);
    else
        % Simple matrix
        m = serialize_numeric_simple(v);
    end
end

% *container* class to byte
function b = class2tag(cls)
	switch cls
		case 'string'
            b = uint8(0);
		case 'double'
			b = uint8(1);
		case 'single'
			b = uint8(2);
		case 'int8'
			b = uint8(3);
		case 'uint8'
			b = uint8(4);
		case 'int16'
			b = uint8(5);
		case 'uint16'
			b = uint8(6);
		case 'int32'
			b = uint8(7);
		case 'uint32'
			b = uint8(8);
		case 'int64'
			b = uint8(9);
		case 'uint64'
			b = uint8(10);
		otherwise
			error('Unknown class');
    end
end
